simulink model "AWES3_CL_wTether_v4_PM"  (R2022a)
settings: Solver=ode3  StartTime=0  StopTime=simInit.TSIM  FixedStep=simInit.dt  RelTol=1e-3
values from neighbouring files (symbols this model uses):
  complex_tether_flag = 1    [run_sim.m]
  Ft_max = 1870    [run_sim.m]
  q = 0    [barrier_optimization.m]
  r = 0    [barrier_optimization.m]
  random_seed = [ 24335       17059       17670        1747]    [run_sim.m]
  safety_controller = false    [run_sim.m]
  turbulence = true    [run_sim.m]
undefined symbols (not defined in the file or in its folder): aeroModel, alpha_max, alpha_min, alpha_options, base_windspeed, constr, DiscIntNeverNeededParam, dx, ENVMT, F, grid_max, grid_min, HDBK, I_table, Light, MIL, mu_max, mu_min, mu_options, P_AP2, params, SampleTime, simInit, T, u0_sim, winchParameter, x0_sim
libraries: simulink x30, aerolibwind2 x14, dspstat3 x2, pid_lib x1, aerolibwindfilters x1, aerolibcommonsys x1, matrix_library x1
(part 5 of 5)

== matlab function AWES3_CL_wTether_v4_PM/FlightController/Retraction/CalculateAttitudeCmds/FlightPathLoopRetraction/inversionPathDynamics ==
  data: flightMode input; nu_chi_a input; mu_a_c output; nu_gamma_a input; P_AP2 parameter; f_t input; pos_O input; chi_a input; gamma_a input; airdata input; constr parameter; alpha_a_c output; ddt_v_w_x_O input; L_rq output; Lrq_old input; mu_a input; mu_a_c_old input; push_mode output; chi_dot_real output; gamma_dot_real output; aeroModel parameter
function [mu_a_c,alpha_a_c,L_rq, push_mode,chi_dot_real,gamma_dot_real] = fcn(flightMode,nu_chi_a, nu_gamma_a,P_AP2, f_t,pos_O, chi_a, gamma_a, airdata, constr, ddt_v_w_x_O, Lrq_old, mu_a,mu_a_c_old, aeroModel)

chi_dot_real = 0;
gamma_dot_real = 0;
push_mode = 0;
mu_a_c = 0;
L_rq = 0;
alpha_a_c = 0;

c_chi_a = cos(chi_a); 
c_gamma_a = cos(gamma_a); 
s_chi_a = sin(chi_a); 
s_gamma_a = sin(gamma_a); 

Va = airdata(1); 
alpha = airdata(2);

M_AbarO = [ c_chi_a*c_gamma_a, s_chi_a*c_gamma_a, -s_gamma_a; 
    -s_chi_a, c_chi_a, 0; 
    c_chi_a*s_gamma_a, s_chi_a*s_gamma_a, c_gamma_a];

F_g_Abar = M_AbarO * [0;0;P_AP2.mass*P_AP2.g];
F_t_Abar = -M_AbarO * pos_O/norm(pos_O)*f_t; 


% if ~wings_level
%     fy  =  P_AP2.mass * ( - sin(chi_a)*ddt_v_w_x_O) - F_g_Abar(2)   ; 
%     fz =   P_AP2.mass  * ( - cos(chi_a)*sin(gamma_a)*ddt_v_w_x_O ) + F_g_Abar(3) ; 
%     %mu_a_c = max( min( atan2(fy,fz), constr.mu_a_max), -constr.mu_a_max); 
%     mu_a_c = tan(gamma_a) * tan( airdata(3) ); % corresponds to PHI = 0 (wings level)
% else
fy  =  P_AP2.mass * ( nu_chi_a * cos(gamma_a) * Va - sin(chi_a)*ddt_v_w_x_O) - F_g_Abar(2) - F_t_Abar(2)  ;
fz =   P_AP2.mass  * (nu_gamma_a * Va              - cos(chi_a)*sin(gamma_a)*ddt_v_w_x_O ) + F_g_Abar(3) + F_t_Abar(3);
mu_a_c = atan2(fy,fz);
% end
push_mode = 0;
L_min =  0.5*P_AP2.rho_air*P_AP2.S_wing*airdata(1)^2 * (aeroModel.CL0+aeroModel.CL_alpha*constr.alpha_a_min); % max. negative lift

% Recalculation of fy, 
%fy = fz * tan(mu_a); % delay in pull-up
fy = fz * tan(mu_a_c); % leads to pitch then bank behavior.

F_req = min( sqrt( fy^2 + fz^2 ), constr.max_lift );

if abs(mu_a_c)>constr.mu_a_max_retraction && abs(F_req)<abs(L_min) || (fz < 0 && flightMode == 6) % in the retraction phase we want to burn tether force hence it makes sense to fly in push mode.
    mu_a_tmp = mu_a_c + pi; 
    if mu_a_tmp > pi
        du = mod(mu_a_tmp,pi);
        mu_a_tmp = -pi+du;
    elseif mu_a_tmp < -pi
        du = mod(mu_a_tmp,-pi);
        mu_a_tmp = pi+du;
    end
    if abs(mu_a_tmp) <= constr.mu_a_max_retraction || flightMode == 6
        mu_a_c = mu_a_tmp;
        push_mode = 1;
    end
end

mu_a_c = max( min( mu_a_c , constr.mu_a_max_retraction), -constr.mu_a_max_retraction);

%fy = fz * max( min( tan(mu_a_c), 1), -1); % first pull up then bank
fy = fz * tan(mu_a_c);

F_req = min( sqrt( fy^2 + fz^2 ), constr.max_lift );

if push_mode
    L_rq = -F_req;
else
    L_rq = F_req;
end

% hold old bank angle if required lift is very small, avoid agressive
% banking for small absolute values of L i.e. for small values inaccuracies
% like numerical inaccuracies have a large impact on the mu_a_c.
if abs(L_rq) <= 1
    mu_a_c = mu_a_c_old;
end

% for large bank angle changes only adapt the lift if close to the current
% lift. The lontitudional dynamic is faster, hence if we command large bank
% angles this would result in a large lift which would first create a large
% curvature in the longi plane before the actual curvature in the lateral
% plan is achieved.
if 0 
if abs( mu_a_c - mu_a ) > constr.max_delta_mu
    L_rq = Lrq_old;
end
end

CL_rq = max( min( 2*L_rq / ( P_AP2.rho_air*P_AP2.S_wing*airdata(1)^2 ), constr.max_CL), constr.min_CL);
alpha_a_c = max( min( (CL_rq-aeroModel.CL0)/aeroModel.CL_alpha, constr.alpha_a_max), constr.alpha_a_min); 
CL = max( min( aeroModel.CL0+aeroModel.CL_alpha*alpha_a_c, constr.max_CL), constr.min_CL);

Lreal = 0.5 * Va^2 * 1.225 * P_AP2.S_wing * CL; 
chi_dot_real = 1/cos(gamma_a)/Va/P_AP2.mass*(sin(mu_a_c)*Lreal + F_g_Abar(2) + F_t_Abar(2));
gamma_dot_real = -1/Va/P_AP2.mass*(-cos(mu_a_c)*Lreal + F_g_Abar(3) + F_t_Abar(3));

== matlab function AWES3_CL_wTether_v4_PM/FlightController/Retraction/CalculateAttitudeCmds/FlightpathReferenceModels/SecondOrderReferenceModel_course/MATLAB Function ==
  data: w0_int output; w0_max input; w0_min input; dynP input; dynP_max input; dynP_min input
function w0_int = fcn(w0_max, w0_min, dynP, dynP_max, dynP_min)

lambda = (dynP - dynP_min)/(dynP_max - dynP_min); 

w0_int = w0_max * lambda + w0_min * (1-lambda);

== matlab function AWES3_CL_wTether_v4_PM/FlightController/Retraction/CalculateAttitudeCmds/FlightpathReferenceModels/SecondOrderReferenceModel_course/calcualteCourseErrorAndWrap ==
  data: chi_ref input; e_course output; chi input
function e_course = fcn(chi_ref, chi)
%#codegen
% The vectors are lying in the tangential plane attached to the current
% position on the small earth.
p_bearing_vec =   [cos(chi);         sin(chi);         0];
p_bearing_vec = p_bearing_vec/norm(p_bearing_vec); 
ref_bearing_vec = [cos(chi_ref); sin(chi_ref); 0];
ref_bearing_vec = ref_bearing_vec/norm(ref_bearing_vec); 

e_z = cross( ref_bearing_vec, p_bearing_vec ); 

dot_product = dot( ref_bearing_vec, p_bearing_vec ); 
if dot_product > 1 
    dot_product = 1; 
end
if dot_product < -1 
    dot_product = -1; 
end

e_course = - sign( e_z(3) ) * acos( dot_product );

if 0 
    1; 
end

== matlab function AWES3_CL_wTether_v4_PM/FlightController/Retraction/CalculateAttitudeCmds/FlightpathReferenceModels/SecondOrderReferenceModel_course/wrap2pi2 ==
  data: u input; y output
function y = fcn(u)
u = mod(u, 2*pi); 
if u > pi 
    du = mod(u,pi);
    y = -pi+du; 
elseif u < -pi 
    du = mod(u,-pi); 
    y = pi+du;
else
    y = u; 
end

== matlab function AWES3_CL_wTether_v4_PM/FlightController/Retraction/CalculateAttitudeCmds/FlightpathReferenceModels/SecondOrderReferenceModel_mu_a/MATLAB Function ==
  data: w0_int output; w0_max input; w0_min input; dynP input; dynP_max input; dynP_min input
function w0_int = fcn(w0_max, w0_min, dynP, dynP_max, dynP_min)

lambda = (dynP - dynP_min)/(dynP_max - dynP_min); 

w0_int = w0_max * lambda + w0_min * (1-lambda);

== matlab function AWES3_CL_wTether_v4_PM/FlightController/Retraction/CalculateAttitudeCmds/FlightpathReferenceModels/SecondOrderReferenceModel_pathangle/MATLAB Function ==
  data: w0_int output; w0_max input; w0_min input; dynP input; dynP_max input; dynP_min input
function w0_int = fcn(w0_max, w0_min, dynP, dynP_max, dynP_min)

lambda = (dynP - dynP_min)/(dynP_max - dynP_min); 

w0_int = w0_max * lambda + w0_min * (1-lambda);

== matlab function AWES3_CL_wTether_v4_PM/FlightController/Retraction/CalculateAttitudeCmds/PIController_opt/wrapCourse ==
  data: chi_ref input; e_course output; chi input
function e_course = fcn(chi_ref, chi)
%#codegen
% The vectors are lying in the tangential plane attached to the current
% position on the small earth.
p_bearing_vec =   [cos(chi);         sin(chi);         0];
p_bearing_vec = p_bearing_vec/norm(p_bearing_vec); 
ref_bearing_vec = [cos(chi_ref); sin(chi_ref); 0];
ref_bearing_vec = ref_bearing_vec/norm(ref_bearing_vec); 

e_z = cross( ref_bearing_vec, p_bearing_vec ); 

dot_product = dot( ref_bearing_vec, p_bearing_vec ); 
if dot_product > 1 
    dot_product = 1; 
end
if dot_product < -1 
    dot_product = -1; 
end

e_course = - sign( e_z(3) ) * acos( dot_product );

if 0 
    1; 
end

== matlab function AWES3_CL_wTether_v4_PM/FlightController/Retraction/CalculateAttitudeCmds/TrafoPathKin2PathAero ==
  data: Vg input; chi_a output; Va input; gamma_k input; chi_k input; v_w_O input; gamma_a output; beta input
function [chi_a, gamma_a] = fcn(Vg, Va, gamma_k,chi_k, v_w_O,  beta)

gamma_a = asin( max( min( (Vg*sin(gamma_k)+v_w_O(3))/(Va+1e-9),1), -1) );
chi_a = beta + chi_k - asin( max( min( 1/(Va*cos(gamma_a)) * (v_w_O(1)*(-sin(chi_k))+v_w_O(2)*cos(chi_k)),1), -1) );
1;
%gamma_a = asin( max( min( (Vg*sin(gamma_k))/(Va+1e-9),1), -1) );
%chi_a = beta + chi_k - asin( max( min( 1/(Va*cos(gamma_a)) ,1), -1) ) ;

== matlab function AWES3_CL_wTether_v4_PM/FlightController/Retraction/GuidanceFlatEarth/MATLAB Function1 ==
  data: vel_k_O input; vel_k_down_W output; vel_k_h_W output; ENVMT parameter
function [vel_k_down_W,vel_k_h_W]   = fcn(vel_k_O,ENVMT)

vel_k_W = transformFromOtoW(ENVMT.windDirection_rad, vel_k_O);

vel_k_h_W = sqrt( vel_k_W(1)^2 + vel_k_W(2)^2 );
vel_k_down_W = vel_k_W(3);

== matlab function AWES3_CL_wTether_v4_PM/FlightController/Retraction/GuidanceFlatEarth/calculateTransitionTrigger1 ==
  data: target_W output; pos_init_retraction_O input; pos_G_O_m input; transition_flag output; ENVMT parameter; vk_xy input; chi_k_cmd output; v_k_tot input; d_horizontal output; d_vertical output; gamma_k_cmd output; constr parameter; params parameter; flag_pos_y_W output; phi0_retraction input; approachFlag output; flare_flag output; Va input
function [target_W, transition_flag, chi_k_cmd, d_horizontal, d_vertical,gamma_k_cmd,flag_pos_y_W, approachFlag, flare_flag] = fcn(pos_init_retraction_O, pos_G_O_m, ENVMT, vk_xy, v_k_tot, constr, params,  phi0_retraction, Va)


pos_init_retraction_W = transformFromOtoW(ENVMT.windDirection_rad, pos_init_retraction_O);

retraction_side = pos_init_retraction_W(2);

if retraction_side > 0
    flag_pos_y_W = 1;
else
    flag_pos_y_W = 0;
end


%% outer point lemniscate
Lbooth.b = params.b_booth;
Lbooth.a = params.b_booth*params.a_booth;
Lbooth.phi0 = phi0_retraction; %80*pi/180;
[Lem] = updateBoothLemniscate(params.l_tether_min,Lbooth);
if flag_pos_y_W
    s = pi/2;
else
    s = 3/2*pi;
end
long_P = Lem.b * sin(s) ./( 1+(Lem.a/Lem.b*cos(s)).^2 );
lat_P =   Lem.a * sin(s).*cos(s) ./ ( 1+(Lem.a/Lem.b*cos(s)).^2 );
p_P = [ cos(long_P).*cos(lat_P);sin(long_P).*cos(lat_P);sin(lat_P)]*params.l_tether_min;
M_WP = [cos(Lbooth.phi0),0, -sin(Lbooth.phi0);0, 1, 0;  sin(Lbooth.phi0),0, cos(Lbooth.phi0)];
p_W = M_WP * p_P;
%%

target_W = p_W;% params.target_retraction_W;
% target_W(2) = p_W(2)-sign( p_W(2) )*10;

% adjust init retraction point for straight glide path
pos_init_retraction_W(2) = target_W(2);


pos_W = transformFromOtoW(ENVMT.windDirection_rad, pos_G_O_m);


switch_WP_x_W = p_W(1);%x_c_W - sin(theta)*r;
switch_WP_y_W = p_W(2);%y_c_W + cos(theta)*r;


switch_WP_W = [switch_WP_x_W;switch_WP_y_W;0];
if ( (pos_W(1) <= p_W(1)+200) && Va<params.vamin ) || (pos_W(1) <= p_W(1))%   %+10;% 20 % 10 works
%if ( (pos_W(1) <= p_W(1)+200) && Va<params.vamin+5 ) || (pos_W(1) <=
%p_W(1))%   % best so far (27.05.2020)
    approachFlag = 1;
else
    approachFlag = 0;
end
%if (pos_W(1) <= p_W(1)) %|| transition_flag_old %pos_W(1) <= switch_WP_x_W || transition_flag_old
if ((pos_W(1) <= p_W(1)+100) && Va<params.vamin) || (pos_W(1) <= p_W(1))%|| transition_flag_old %pos_W(1) <= switch_WP_x_W || transition_flag_old
    transition_flag = 1;
else
    transition_flag = 0;
end

%% Reference Course Calculation
groundtrack_bearing_W = target_W - pos_init_retraction_W;
groundtrack_bearing_O = transformFromWtoO(ENVMT.windDirection_rad, groundtrack_bearing_W);
chi_k_cmd = atan2( groundtrack_bearing_O(2), groundtrack_bearing_O(1) );
groundtrack_bearing_W(3) = 0;
pos_rel_gt_W = pos_W - pos_init_retraction_W;
pos_rel_gt_W(3) = 0;
p_proj_W = pos_rel_gt_W'*groundtrack_bearing_W / norm( groundtrack_bearing_W )^2 * groundtrack_bearing_W;
d_horizontal = norm( pos_rel_gt_W - p_proj_W );
z = cross( groundtrack_bearing_W,pos_rel_gt_W );
delta_chi = sign(z(3)) * asin( max( min( 2*params.kp_delta_course*d_horizontal / vk_xy, 1),-1) );
chi_k_cmd = chi_k_cmd + delta_chi;

%% Reference Descend Angle Calculation
z_transition = sqrt( params.l_tether_min^2 - switch_WP_x_W^2 - switch_WP_y_W^2 ); % min. attitude has higher priority then min. tether length
dh = pos_init_retraction_W(3) - z_transition;
ds = sqrt( ( switch_WP_x_W - pos_init_retraction_W(1))^2 +  ( switch_WP_y_W - pos_init_retraction_W(2))^2 );
gamma_k_star =  -atan( dh/ds );
gs_direction_W = [switch_WP_W(1) - pos_init_retraction_W(1);switch_WP_W(2) - pos_init_retraction_W(2);-dh];
p_rel_W = pos_W - pos_init_retraction_W;
p_proj_W = p_rel_W'*gs_direction_W / norm( gs_direction_W )^2 * gs_direction_W;
d_vertical = norm( p_rel_W(3) - p_proj_W(3) );
z = cross( gs_direction_W,p_rel_W );
sign_deltaGamma = sign(z(2));
gamma_k_cmd = gamma_k_star - asin( max( min(params.kp_delta_gamma*d_vertical*sign_deltaGamma/(v_k_tot+1e-3), pi/6), -pi/6) );

%% Potential flare maneuver 
gamma_k_cmd_tmp = gamma_k_cmd;
x0 = 50; % flare range
g_f = 10*pi/180;
if (pos_W(1) < (x0+target_W(1)))&& Va>params.vamin
    flare_flag = 0;
    b = log( g_f - gamma_k_star + 1 )/x0;
    gamma_k_cmd = max( min( gamma_k_star + max( exp( - ( pos_W(1) -  target_W(1) - x0)*b ) - 1, 0 ), g_f ), gamma_k_cmd_tmp );
else
    flare_flag = 0;
end

== matlab function AWES3_CL_wTether_v4_PM/FlightController/Traction/FlightPathLoopTraction/EstimatePlantResponse/MATLAB Function ==
  data: dphi input; mu_k input; chi_dot_real output; gamma_dot_real output; P_AP2 parameter; chi_k input; gamma_k input; F_t input; pos_O input; v_k_B input; airdata input; aeroModel parameter
function [chi_dot_real, gamma_dot_real] = fcn(dphi, mu_k,P_AP2,chi_k,gamma_k, F_t, pos_O, v_k_B, airdata, aeroModel)

Va = airdata(1); 
alpha = airdata(2); 
vk = norm(v_k_B); 
%CL = max( min( aero_ctrl.CL_0 + aero_ctrl.dCLdalpha*alpha, aero_ctrl.clmax), aero_ctrl.clmin ); 
CL = aeroModel.CL0 + aeroModel.CL_alpha*alpha; 

Lrq = 0.5 * Va^2 * 1.225 * P_AP2.S_wing * CL; 


c_chi_k = cos(chi_k); 
c_gamma_k = cos(gamma_k); 
s_chi_k = sin(chi_k); 
s_gamma_k = sin(gamma_k); 


M_KO = [ c_chi_k*c_gamma_k, s_chi_k*c_gamma_k, -s_gamma_k; 
    -s_chi_k, c_chi_k, 0; 
    c_chi_k*s_gamma_k, s_chi_k*s_gamma_k, c_gamma_k];

F_g_t_K = M_KO * ( [0;0;P_AP2.mass*P_AP2.g] -F_t*pos_O/norm(pos_O) );
% 
% v_a_B = [cos(alpha_sat)*cos(beta); 
%         sin(beta);
%         sin(alpha_sat)*cos(beta)]*Va;
%     
% v_k_B = v_a_B + v_w_B_hat; 
% 
% alpha_k_sat = atan2( v_k_B(3), v_k_B(1) ); 
% beta_k = asin( v_a_B(2)/norm(v_k_B) ); 
%     
% M_KB = [ cos(alpha_k_sat)*cos(beta_k), sin(beta_k), sin(alpha_k_sat)*cos(beta_k);
%     -cos(alpha_k_sat)*sin(beta_k)*cos(mu_k) + sin(alpha_k_sat)*sin(mu_k), cos(beta_k)*cos(mu_k), -sin(alpha_k_sat)*sin(beta_k)*cos(mu_k)-sin(mu_k)*cos(alpha_k_sat);
%     -cos(alpha_k_sat)*sin(beta_k)*sin(mu_k) - sin(alpha_k_sat) * cos(mu_k),cos(beta_k)*sin(mu_k),-sin(alpha_k_sat)*sin(beta_k)*sin(mu_k)+cos(alpha_k_sat)*cos(mu_k)];

%F_a_K_est = M_KB * F_a_B_est; 

%chi_dot_real = 1/cos(gamma_k)/norm(v_k_B)/P_AP2.mass  * ( F_a_K_est(2) + F_g_t_K(2) );
%gamma_dot_real = -1/norm(v_k_B)/P_AP2.mass * ( F_a_K_est(3) + F_g_t_K(3) );

f_bar_z_K = -Lrq/sqrt(1+(tan(mu_k-dphi))^2); 
%if mu_k >= 0 
 %   f_bar_y_K = sqrt( Lrq^2 - (Lrq/sqrt(1+(tan(mu_k-dphi))^2))^2 ); 
%else
 %   f_bar_y_K = -sqrt( Lrq^2 - (Lrq/sqrt(1+(tan(mu_k-dphi))^2))^2 ); 
%end
f_bar_y_K = -f_bar_z_K * tan( mu_k - dphi );

%chi_dot_real = 1/cos(gamma_k)/norm(v_k_B)/P_AP2.mass  * ( F_a_K_est(2) + F_g_t_K(2) );
%gamma_dot_real = -1/norm(v_k_B)/P_AP2.mass * ( F_a_K_est(3) + F_g_t_K(3) );
chi_dot_real = 1/cos(gamma_k)/vk/P_AP2.mass  * ( f_bar_y_K + F_g_t_K(2) );
gamma_dot_real = -1/vk/P_AP2.mass * ( f_bar_z_K + F_g_t_K(3) );

== matlab function AWES3_CL_wTether_v4_PM/FlightController/Traction/FlightPathLoopTraction/MATLAB Function ==
  data: L_rq output; airdata input; P_AP2 parameter
function L_rq = fcn(airdata, P_AP2)

L_rq =  min( 0.5*P_AP2.rho_air*P_AP2.S_wing*airdata(1)^2 * (P_AP2.CL0+P_AP2.CL_alpha*airdata(2) ),1800); % max. negative lift

== matlab function AWES3_CL_wTether_v4_PM/FlightController/Traction/FlightPathLoopTraction/inversionPathDynamics ==
  data: Ft_set input; nu_chi_k input; mu_a output; nu_gamma_k input; F_a_B_est input; P_AP2 parameter; pos_O input; chi_k input; gamma_k input; v_k_B input; pathangles_a input; airdata input; constr parameter; mu_k_c output; alpha_rq output; dphi output; L_rq output; L_rq_old input; mu_a_old input; aeroModel parameter
 function [mu_a,mu_k_c,alpha_rq,dphi,L_rq] = fcn(  Ft_set,nu_chi_k, nu_gamma_k, F_a_B_est,P_AP2,pos_O,...
     chi_k, gamma_k, v_k_B, pathangles_a, airdata,constr, L_rq_old, mu_a_old, aeroModel)
fbar_z_K = 0;
mu_a = 0;
mu_k_c = 0;
alpha_rq = 0;
dphi = 0;
v_k = 0;
L_rq = 0;
fbar_z_K = 0;
fbar_z_K_is = 0;

chi_a = pathangles_a(1);
gamma_a = pathangles_a(2);

f_t = Ft_set; 
mu_k_max = constr.mu_k_max;

beta_a = airdata(3); 

alpha_k = asin( v_k_B(3)/norm(v_k_B) ); 
beta_k = atan2( v_k_B(2), v_k_B(1) ); 

v_k = norm(v_k_B); 

c_chi_k = cos(chi_k); 
c_gamma_k = cos(gamma_k); 
s_chi_k = sin(chi_k); 
s_gamma_k = sin(gamma_k); 

% c_chi_a = cos(chi_a); 
% c_gamma_a = cos(gamma_a); 
% s_chi_a = sin(chi_a); 
% s_gamma_a = sin(gamma_a); 

M_KO = [ c_chi_k*c_gamma_k, s_chi_k*c_gamma_k, -s_gamma_k; 
    -s_chi_k, c_chi_k, 0; 
    c_chi_k*s_gamma_k, s_chi_k*s_gamma_k, c_gamma_k];
% 
% M_AbarO = [ c_chi_a*c_gamma_a, s_chi_a*c_gamma_a, -s_gamma_a; 
%     -s_chi_a, c_chi_a, 0; 
%     c_chi_a*s_gamma_a, s_chi_a*s_gamma_a, c_gamma_a];
% 
% M_AbarK = M_AbarO*M_KO';


f_a_x_B = F_a_B_est(1); 
f_a_y_B = F_a_B_est(2); 
f_a_z_B = F_a_B_est(3); 


f_a_y_Kbar = -cos(alpha_k)*sin(beta_k)*f_a_x_B + cos(beta_k)*f_a_y_B - sin(alpha_k)*sin(beta_k)*f_a_z_B; 
f_a_z_Kbar = -sin(alpha_k)*f_a_x_B + cos(alpha_k)*f_a_z_B; 

f_t_K = -M_KO * pos_O/norm(pos_O)*f_t; 

%fbar_x_K = 0*P_AP2.mass*a_tot + sin(gamma_k)*P_AP2.mass*P_AP2.g - f_t_K(1);
fbar_y_K = P_AP2.mass*nu_chi_k*cos(gamma_k)*v_k - f_t_K(2); 
fbar_z_K = -P_AP2.mass*nu_gamma_k*v_k - cos(gamma_k)*P_AP2.mass*P_AP2.g - f_t_K(3);

% % contributions
% ft_contribution_fy = -f_t_K(2);
% ft_contribution_fz = f_t_K(3);
% rest_contribution_fy = -P_AP2.mass*nu_chi_k*cos(gamma_k)*v_k;
% rest_contribution_fz = -P_AP2.mass*nu_gamma_k*v_k - cos(gamma_k)*P_AP2.mass*P_AP2.g;
% 
% contributions_tot = [ft_contribution_fy, ft_contribution_fz, rest_contribution_fy, rest_contribution_fz];

%F_c_K = [fbar_x_K;fbar_y_K;fbar_z_K];
%  constraint already here the commanded force
% if f_a_k_limit_1 >= f_a_k_limit_2
%     f_max =  f_a_k_limit_1;
%     f_min = f_a_k_limit_2;
% else
%     f_max =  f_a_k_limit_2;
%     f_min = f_a_k_limit_1;
% end
% 
% if fbar_z_K >= f_max 
%     fbar_z_K = f_max;
% elseif fbar_z_K <= f_min
%     fbar_z_K = f_min;
% end

dphi = 0 * atan( f_a_y_Kbar / f_a_z_Kbar ); % this might be important at high wind speeds
% if abs(f_a_y_Kbar) < 1e-12
%    mu_k_c = atan2( fbar_y_K,  -fbar_z_K);
%    fbar_y_K = -tan(mu_k_c)*fbar_z_K;
%     dphi = 0; 
% elseif


%if abs(f_a_z_Kbar) < 1e-12
 %   mu_k_c = atan2( fbar_z_K,  fbar_y_K);
  %  fbar_y_K = tan(mu_k_c)*fbar_y_K; % enables first pullup then bank behavior
%else
   mu_k_c = atan2( fbar_y_K, -fbar_z_K ) + dphi; 
   fbar_y_K =  -fbar_z_K * tan( mu_k_c - dphi );
%end

%L_rq = min( sqrt( fbar_y_K^2 + fbar_z_K^2 ), 1800); % constraint by max. tether force e.g. structural limit
L_rq = min( sqrt( fbar_y_K^2 + fbar_z_K^2 )); % constraint by max. tether force e.g. structural limit

%F_c_Abar = M_AbarK * F_c_K;

%mu_a_c_correct = atan2( F_c_Abar(2), F_c_Abar(3) );

%L_rq_correct = sqrt( F_c_Abar(2)^2 + F_c_Abar(3)^2 );

%L_rq = L_rq_correct;

mu_k_pre_sat = mu_k_c; 
% limit mu_k: We do this for now directly: if we assume that the kite is in
% the tangential plane this corresponds well to the limits for phi_tau

%if flightMode == 10
 %   mu_k_max = 30*pi/180;
%    mu_k_c = max( min( mu_k_c, mu_k_max), -mu_k_max); 
%else
    mu_k_c = max( min( mu_k_c, mu_k_max), -mu_k_max); 
%end

% % constraining additionally over max. phi_tau
% phi_tau_c = asin( max(min(cos(beta_k)/cos(eta_tau_rad(2)) * sin(mu_k_c),1),-1) );
% phi_tau_c_max =  80*pi/180;
% if phi_tau_c > phi_tau_c_max
%     mu_k_c = asin( max( min( sin(phi_tau_c_max) *  cos(eta_tau_rad(2)) / cos(beta_k), 1),-1) ); 
% elseif phi_tau_c < -phi_tau_c_max
%     mu_k_c = asin( sin(-phi_tau_c_max) *  cos(eta_tau_rad(2)) / cos(beta_k) ); 
% end  

% Go over the tangential plane frame: Allow limitation of mu_a through
% limits on phi_tau!
%phi_tau = asin(  max( min((sin(mu_k_c))*cos(beta_k), 1),-1) ); 
% TO-DO: Restrict roll-angle with respect to tangential plane: 
% calculate first phi_tau, then limit phi_tau, then calculate phi from
% phi_tau and use this for the calculation of mu_a
if 0
    phi = asin(  max( min((sin(mu_k_c)-tan(gamma_k)*tan(beta_k)) * cos(gamma_k)*cos(beta_k), 1),-1) );
    mu_a = asin(  max( min(sin(phi)/cos(gamma_a)/cos(beta_a)  + tan(gamma_a)*tan(beta_a) , 1),-1)  );
else
    mu_a = mu_k_c;
end
%mu_a = asin(  max( min(sin(phi)*cos(eta_OB_rad(2))/cos(gamma_a)/cos(beta_a)  + tan(gamma_a)*tan(beta_a) , 1),-1)  ); 

% hold old bank angle if required lift is very small, avoid agressive
% banking for small absolute values of L i.e. for small values inaccuracies
% like numerical inaccuracies have a large impact on the mu_a_c.
if abs(L_rq) <= 10
   % mu_a = mu_a_old;
end

% for large bank angle changes only adapt the lift if close to the current
% lift. The longitudional dynamic is faster, hence if we command large bank
% angles this would result in a large lift which would first create a large
% curvature in the longi plane before the actual curvature in the lateral
% plan is achieved.
if abs( mu_a - mu_a_old ) > constr.max_delta_mu
   % L_rq = L_rq_old;
end

CL_rq = 2*L_rq / ( P_AP2.rho_air*P_AP2.S_wing*airdata(1)^2 );
alpha_rq = (CL_rq - aeroModel.CL0)/aeroModel.CL_alpha;

== matlab function AWES3_CL_wTether_v4_PM/FlightController/Traction/FlightPathLoopTraction/inversionPathDynamics1 ==
  data: Ft_set input; nu_chi_k input; mu_a output; nu_gamma_k input; F_a_B_est input; P_AP2 parameter; pos_O input; chi_k input; gamma_k input; v_k_B input; gamma_a input; airdata input; constr parameter; mu_k_c output; alpha_rq output; dphi output; L_rq output; L_rq_old input; mu_a_old input
 function [mu_a,mu_k_c,alpha_rq,dphi,L_rq] = fcn(  Ft_set,nu_chi_k, nu_gamma_k, F_a_B_est,P_AP2,pos_O,...
     chi_k, gamma_k, v_k_B, gamma_a, airdata,constr, L_rq_old, mu_a_old)
fbar_z_K = 0;
mu_a = 0;
mu_k_c = 0;
alpha_rq = 0;
dphi = 0;
v_k = 0;
L_rq = 0;
fbar_z_K = 0;
fbar_z_K_is = 0;

f_t = Ft_set; 
mu_k_max = constr.mu_k_max;

beta_a = airdata(3); 

alpha_k = asin( v_k_B(3)/norm(v_k_B) ); 
beta_k = atan2( v_k_B(2), v_k_B(1) ); 

v_k = norm(v_k_B); 

c_chi_k = cos(chi_k); 
c_gamma_k = cos(gamma_k); 
s_chi_k = sin(chi_k); 
s_gamma_k = sin(gamma_k); 

M_KO = [ c_chi_k*c_gamma_k, s_chi_k*c_gamma_k, -s_gamma_k; 
    -s_chi_k, c_chi_k, 0; 
    c_chi_k*s_gamma_k, s_chi_k*s_gamma_k, c_gamma_k];

f_a_x_B = F_a_B_est(1); 
f_a_y_B = F_a_B_est(2); 
f_a_z_B = F_a_B_est(3); 


f_a_y_Kbar = -cos(alpha_k)*sin(beta_k)*f_a_x_B + cos(beta_k)*f_a_y_B - sin(alpha_k)*sin(beta_k)*f_a_z_B; 
f_a_z_Kbar = -sin(alpha_k)*f_a_x_B + cos(alpha_k)*f_a_z_B; 

f_t_K = -M_KO * pos_O/norm(pos_O)*f_t; 

fbar_y_K = P_AP2.mass*nu_chi_k*cos(gamma_k)*v_k - f_t_K(2); 
fbar_z_K = -P_AP2.mass*nu_gamma_k*v_k - cos(gamma_k)*P_AP2.mass*P_AP2.g - f_t_K(3);

%  constraint already here the commanded force
% if f_a_k_limit_1 >= f_a_k_limit_2
%     f_max =  f_a_k_limit_1;
%     f_min = f_a_k_limit_2;
% else
%     f_max =  f_a_k_limit_2;
%     f_min = f_a_k_limit_1;
% end
% 
% if fbar_z_K >= f_max 
%     fbar_z_K = f_max;
% elseif fbar_z_K <= f_min
%     fbar_z_K = f_min;
% end

dphi = atan( f_a_y_Kbar / f_a_z_Kbar ); % this might be important at high wind speeds
% if abs(f_a_y_Kbar) < 1e-12
%    mu_k_c = atan2( fbar_y_K,  -fbar_z_K);
%    fbar_y_K = -tan(mu_k_c)*fbar_z_K;
%     dphi = 0; 
% elseif
if abs(f_a_z_Kbar) < 1e-12
    mu_k_c = atan2( fbar_z_K,  fbar_y_K);
    fbar_y_K = tan(mu_k_c)*fbar_y_K; % enables first pullup then bank behavior
else
   mu_k_c = atan2( fbar_y_K, -fbar_z_K ) + dphi; 
   fbar_y_K =  -fbar_z_K * tan( mu_k_c - dphi );
end

%L_rq = min( sqrt( fbar_y_K^2 + fbar_z_K^2 ), 1800); % constraint by max. tether force e.g. structural limit
L_rq = min( sqrt( fbar_y_K^2 + fbar_z_K^2 )); % constraint by max. tether force e.g. structural limit

mu_k_pre_sat = mu_k_c; 
% limit mu_k: We do this for now directly: if we assume that the kite is in
% the tangential plane this corresponds well to the limits for phi_tau
mu_k_c = max( min( mu_k_c, mu_k_max), -mu_k_max); 

% % constraining additionally over max. phi_tau
% phi_tau_c = asin( max(min(cos(beta_k)/cos(eta_tau_rad(2)) * sin(mu_k_c),1),-1) );
% phi_tau_c_max =  80*pi/180;
% if phi_tau_c > phi_tau_c_max
%     mu_k_c = asin( max( min( sin(phi_tau_c_max) *  cos(eta_tau_rad(2)) / cos(beta_k), 1),-1) ); 
% elseif phi_tau_c < -phi_tau_c_max
%     mu_k_c = asin( sin(-phi_tau_c_max) *  cos(eta_tau_rad(2)) / cos(beta_k) ); 
% end  

% Go over the tangential plane frame: Allow limitation of mu_a through
% limits on phi_tau!
%phi_tau = asin(  max( min((sin(mu_k_c))*cos(beta_k), 1),-1) ); 
% TO-DO: Restrict roll-angle with respect to tangential plane: 
% calculate first phi_tau, then limit phi_tau, then calculate phi from
% phi_tau and use this for the calculation of mu_a
phi = asin(  max( min((sin(mu_k_c)-tan(gamma_k)*tan(beta_k)) * cos(gamma_k)*cos(beta_k), 1),-1) ); 
mu_a = asin(  max( min(sin(phi)/cos(gamma_a)/cos(beta_a)  + tan(gamma_a)*tan(beta_a) , 1),-1)  ); 
%mu_a = asin(  max( min(sin(phi)*cos(eta_OB_rad(2))/cos(gamma_a)/cos(beta_a)  + tan(gamma_a)*tan(beta_a) , 1),-1)  ); 

% hold old bank angle if required lift is very small, avoid agressive
% banking for small absolute values of L i.e. for small values inaccuracies
% like numerical inaccuracies have a large impact on the mu_a_c.
if abs(L_rq) <= 10
    mu_a = mu_a_old;
end

% for large bank angle changes only adapt the lift if close to the current
% lift. The longitudional dynamic is faster, hence if we command large bank
% angles this would result in a large lift which would first create a large
% curvature in the longi plane before the actual curvature in the lateral
% plan is achieved.
if abs( mu_a - mu_a_old ) > constr.max_delta_mu
    L_rq = L_rq_old;
end

CL_rq = 2*L_rq / ( P_AP2.rho_air*P_AP2.S_wing*airdata(1)^2 );
alpha_rq = (CL_rq - P_AP2.CL0)/P_AP2.CL_alpha;

== matlab function AWES3_CL_wTether_v4_PM/FlightController/Traction/Navigator/LissajousFigure8Following ==
  data: Delta_chi_dot output; pos_W input; v_w_vec input; v_O_vec input; ENVMT parameter; p_C_W output; sol output; c0 input; lat input; long input; chi_tau output; chi_tau_dot_predict output; chi_tau_is output; chi_k_ideal output; gamma_k_ideal output; params parameter; pathAngles input; gamma_tau_dot input; gamma_tau_cmd input; gamma_tau_is output; chi_dot output; gamma_dot output; PHI_BOOTH input; delta_ct output; delta0 output; delta_ct_signed output; pathRotFlag input
function [Delta_chi_dot, p_C_W, sol,chi_tau,chi_tau_dot_predict, chi_tau_is, chi_k_ideal, gamma_k_ideal, gamma_tau_is,chi_dot, gamma_dot, delta_ct,delta0, delta_ct_signed] = ...
    fcn(pos_W,v_w_vec, v_O_vec, ENVMT, c0, lat, long,params,pathAngles,gamma_tau_dot,gamma_tau_cmd, PHI_BOOTH, pathRotFlag)
% =========================================================================
% Version: 1.0.
% Author: Sebastian Rapp
% Mail: s.rapp@tudelft.nl
% Unlinke the other modules this module directly calculates the desired
% course and path angle rate
% =========================================================================
windDirection_rad = ENVMT.windDirection_rad;
%v_w_vec = transformFromOtoW( windDirection_rad, v_O_vec); 
b_booth = params.b_booth;
a_booth = params.a_booth;
%PHI_BOOTH = params.phi0_booth;
% 
if pathRotFlag
    Vmax = 60;
else
    Vmax = 60; % 10;15;20;
end
v_w_vec_tot = min(  norm( v_w_vec ), Vmax ); 
v_w_vec = v_w_vec/norm( v_w_vec )*v_w_vec_tot; 
v_O_vec = transformFromWtoO( windDirection_rad, v_w_vec ); 
% total kinematic velocity
Vtot = sqrt( v_O_vec'*v_O_vec );
% 
% if ~pathRotFlag
%     gamma_tau_cmd = -10*pi/180; 
% end



% transform position from NEDframe (O) into Windframe (W)
%pos_W = transformFromOtoW( windDirection_rad, pos_O );
phi_p_mean = PHI_BOOTH;  
M_WP = [cos(phi_p_mean),0, -sin(phi_p_mean);0, 1, 0; sin(phi_p_mean),0, cos(phi_p_mean)];
pos_P = M_WP' * pos_W; 

distanceOrigin = norm(pos_P);

% ------ I think here the curve dependent part starts
if 0 % lissajous
    % Step 0: Update Lissajous figure
%     [ LemPs ] = updateLissajous( distanceOrigin, LemPsRef );
%     direction = -1;
%     % Step 1: Determine closest point
%     [  sol,p_C_W] = getTargetOnLissajousNewton(LemPs, pos_W, c0, distanceOrigin, direction);
%     [t,DtDs,L,dLds,q] = getPathInfos(sol,LemPs, direction);
else % Booth Lemniscate
   % Lbooth.phi0 = PHI_BOOTH;
    Lbooth.a = a_booth*b_booth; % height
    Lbooth.b = b_booth; % length
    Lbooth.phi0 = PHI_BOOTH; %phi0_booth*pi/180;
    % Adapt phi0 -> flight with constant height
 
    [Lem] = updateBoothLemniscate(distanceOrigin,Lbooth);
    direction = params.direction;
    [ sol,p_C_P] = getTargetOnBoothNewton2(Lem, pos_P, c0, distanceOrigin, direction);
    [t_P,DtDs_P,L,dLds,q] = getBoothInfos2(sol,Lem, direction);
    t = M_WP * t_P; 
    DtDs = M_WP * DtDs_P; 
    p_C_W = M_WP * p_C_P; 

    %[ sol,p_C_W] = getTargetOnBoothNewton(Lem, pos_W, c0, distanceOrigin, direction);
    %[t,DtDs,L,dLds,q] = getBoothInfos(sol,Lem, direction);
end    

% ---- I Think everything below is curve independent -----

% Step 2: Calculate distance to closest point
delta = acos( min( max( pos_W'/norm(pos_W) * p_C_W/norm(p_C_W), -1),1 ) );% * norm(pos_W);
delta_ct = delta * distanceOrigin;

% Step 3: Calculate the perpendicular course
[ perpCourse, delta_vec, bearing_sign ] = calcCourse2ClosestPoint( p_C_W, pos_W );
delta_ct_signed = bearing_sign*delta;

% Step 3.5: Parallel transport of vectors at the path point to the kite
% position
t_rot = doRodriguesRotation(pos_W, p_C_W, t);
t_rot_T = transformFromWtoTau(long, lat, t_rot);
chi_parallel = atan2( t_rot_T(2), t_rot_T(1) );

chi = atan2( v_O_vec(2), v_O_vec(1) ); 
gamma = -asin( v_O_vec(3)/norm(v_O_vec) ); 
bearing_is_O = [cos(chi)*cos(gamma);
    sin(chi)*cos(gamma);
    -sin(gamma)];
bearing_is_tau = transformFromWtoTau( long, lat, transformFromOtoW(windDirection_rad, bearing_is_O));
chi_tau_is = atan2( bearing_is_tau(2), bearing_is_tau(1));
gamma_tau_is = -asin( bearing_is_tau(3) / norm( bearing_is_tau ) );

% Step 4: Calculate commanded course in tangential plane
% and determine the ideal bearing vector
%delta0 = tau;%norm(v_w_vec/norm(pos_W)) * tau;
%kp = 100; 
V_k_tau = [cos(chi_tau_is)*cos(gamma_tau_is),sin(chi_tau_is)*cos(gamma_tau_is),0]*Vtot/distanceOrigin; 
% delta0 = 10;% kp/norm(V_k_tau);  
delta0 = min(params.delta0_slope*norm(V_k_tau),0.1)+params.delta0_offset;%0.0025*max( min( norm(V_k_tau), 35),25) ;
% if ~pathRotFlag
%    delta0 = delta0*10; 
% else
%     1;
% end
%delta0 = delta0_in; 
%tau = 1;
%delta0 = norm(v_w_vec/norm(pos_W)) * tau;

[chi_tau, Delta_chi,theta, Delta_chi_dot, deltaDot1] = calculateCommandedCourse2(t_rot,delta_vec, delta, delta0, chi_parallel, p_C_W, pos_W,v_w_vec, chi_tau_is);
%gamma_tau = 10*pi/180;
%v_tau = [cos(chi_tau); sin(chi_tau); 0]*Vtot;

% Step 5: Predict the required course rate due to the path curvature
[chi_tau_dot_predict] = predictChiDotRequ(long,lat,v_w_vec, pos_W,p_C_W, t, DtDs,chi_parallel );

%gamma_tau = max(gamma_tau_dot, gamma_tau_is);%gamma_tau_cmd;%0*gamma_tau_is + delta_gamma_tau;
gamma_tau = gamma_tau_cmd;%gamma_tau_is;%gamma_tau_cmd;%0*gamma_tau_is + delta_gamma_tau;
%gamma_tau = gamma_tau_is;

v_tau = [cos(chi_tau)*cos(gamma_tau); 
         sin(chi_tau)*cos(gamma_tau); 
        -sin(gamma_tau)]*Vtot;
%v_tau = [cos(chi_tau)*cos(gamma_tau); sin(chi_tau)*cos(gamma_tau); v_z_tau/Vtot]*Vtot;

v_w_vec_ideal = transformFromTautoW(long,lat, v_tau);
bearing_O = transformFromWtoO(windDirection_rad, v_w_vec_ideal); 
chi_k_ideal = atan2( bearing_O(2), bearing_O(1) ); 
gamma_k_ideal = -asin( bearing_O(3)/norm(bearing_O) ); 

% Step 6: Calculate current course error for feedback part
%chi = atan2( v_O_vec(2), v_O_vec(1) ); 
%gamma = -asin( v_O_vec(3)/norm(v_O_vec) ); 
%e_chi_tau = wrapCourseError( chi_tau,chi_tau_is);
%e_gamma_tau = gamma_tau - gamma_tau_is;

% Step 7: Calculate the required course rate in the tangential plane 
%chi_tau_dot_cmd = chi_tau_dot_predict + Delta_chi_dot + Kp_chi*e_chi;
%if pathRotFlag
    nu_ref = chi_tau_dot_predict + Delta_chi_dot* pathRotFlag;
%else
 %  nu_ref = chi_tau_dot_predict;  
%end
%%
%long = longlat(1); 
%lat = longlat(2); 
chi = pathAngles(1); 
gamma = pathAngles(2);
chi_tau_dot_cmd = nu_ref ;
%pos_W = transformFromOtoW(ENVMT.windDirection_rad, pos_O); 
[chi_dot, gamma_dot] = getChiDotGammaDotOK(ENVMT.windDirection_rad,lat,long, v_w_vec,...
    chi_tau_dot_cmd, norm(pos_W),chi, gamma, v_w_vec_ideal, pos_W,gamma_tau,gamma_tau_dot);

== matlab function AWES3_CL_wTether_v4_PM/FlightController/Traction/Navigator/calcualteCourseErrorAndWrap1 ==
  data: chi_ref input; e_course output; chi input
function e_course = fcn(chi_ref, chi)
%#codegen
% The vectors are lying in the tangential plane attached to the current
% position on the small earth.
p_bearing_vec =   [cos(chi);         sin(chi);         0];
p_bearing_vec = p_bearing_vec/norm(p_bearing_vec); 
ref_bearing_vec = [cos(chi_ref); sin(chi_ref); 0];
ref_bearing_vec = ref_bearing_vec/norm(ref_bearing_vec); 

e_z = cross( ref_bearing_vec, p_bearing_vec ); 

dot_product = dot( ref_bearing_vec, p_bearing_vec ); 
if dot_product > 1 
    dot_product = 1; 
end
if dot_product < -1 
    dot_product = -1; 
end

e_course = - sign( e_z(3) ) * acos( max(min(dot_product,1),-1) );

if 0 
    1; 
end

== matlab function AWES3_CL_wTether_v4_PM/Visualization/MATLAB Function3 ==
  data: lat input; y output; long input; z input; ENVMT parameter; pos_O output
function [y, pos_O] = fcn(lat, long,z,ENVMT )
windDirection_rad = ENVMT.windDirection_rad; 
M_OW = [cos(windDirection_rad), sin(windDirection_rad), 0;
    sin(windDirection_rad), -cos(windDirection_rad), 0;
    0, 0, -1];

pos_W = [cos(lat)*cos(long); cos(lat)*sin(long); sin(lat)]*z; 
%pos_O = transformFromWtoO(windDirection_rad, pos_W);
pos_O = M_OW*pos_W; 


y = pos_W;

== stateflow chart AWES3_CL_wTether_v4_PM/FlightController/Retraction/GuidanceFlatEarth/Chart ==
  state speedbypitch1 [commented out]
    during: speed_by_pitch =1;
  state Default
    during: speed_by_pitch = 0;
  state speedbypitch
    during: speed_by_pitch =1;
  Default -> speedbypitch1 [commented out] : [va>vamax]
  speedbypitch1 -> Default [commented out] : [va<vamax_min]
  Default -> speedbypitch : [va<vamin && flare_flag == 0]
  (default) -> Default
  speedbypitch -> Default : [va>vamin_max || flare_flag == 1]
  data: flare_flag input; va input; vamin_max parameter; speed_by_pitch output; vamin parameter; vamax_min parameter; vamax parameter
